simulink model "simulink5ms_plotAndGains"  (R2023a)
settings: Solver=ode3  StartTime=0.0  StopTime=1000  FixedStep=.001  RelTol=1e-3  EnableMultiTasking=on
undefined symbols (not defined in the file or in its folder): Serial_Port, Standard_Devices
libraries: sldrtlib x2
settings Model: SimulationMode=external  ExtModeTrigDuration=10000  Creator=d-block  LastModifiedBy=rout3
settings SolverCC: AlgebraicLoopSolver=TrustRegion
settings DataIOCC: LimitDataPoints=on  SaveFormat=Array  ReturnWorkspaceOutputs=off
settings OptimizationCC: LifeSpan=inf
settings DebuggingCC: UnconnectedInputMsg=warning  UnconnectedOutputMsg=warning  UnconnectedLineMsg=warning  SFUnexpectedBacktrackingDiag=warning  SFNoUnconditionalDefaultTransitionDiag=warning  ArithmeticOperatorsInVariantConditions=warning
settings HardwareCC: ProdBitPerLong=64  ProdHWDeviceType=Intel->x86-64 (Linux 64)  TargetBitPerLong=64  TargetBitPerPointer=64  TargetIntDivRoundTo=Zero  TargetEndianess=LittleEndian  TargetWordSize=64  TargetHWDeviceType=Intel->x86-64
settings ModelReferenceCC: EnableRefExpFcnMdlSchedulingChecks=on  PropagateSignalLabelsOutOfModel=off
settings SFSimCC: SimUseLocalCustomCode=off  CustomCodeUndefinedFunction=UseInterfaceOnly
settings RTWCC: Description=Simulink Desktop Real-Time  SystemTargetFile=sldrt.tlc  TemplateMakefile=sldrt.tmf  RTWUseLocalCustomCode=off  RTWCompilerOptimization=on  DLArmComputeVersion=19.05
settings CodeAppCC: MaxIdLength=95  StateflowObjectComments=on
settings SimulinkDesktopRealTimeCC: TargetLibSuffix=_sldrt.a  TargetPreCompLibLocation=C:\MATLABR2023a\toolbox\sldrt\lib\win64  TargetLangStandard=C89/C90 (ANSI)  SupportVariableSizeSignals=off
settings ConfigComp: CovMetricSettings=dw  CovSaveCumulativeToWorkspaceVar=on  CovSaveSingleToWorkspaceVar=on  CovExternalEMLEnable=off

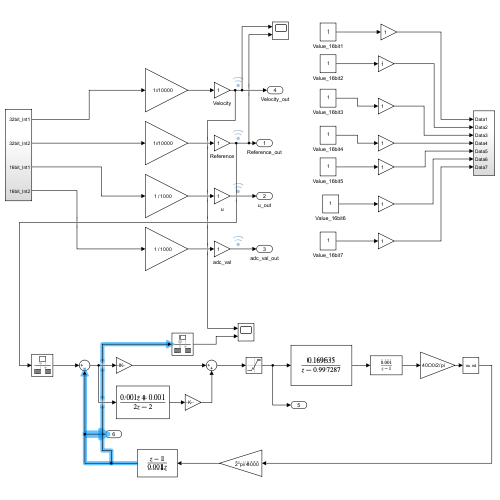
[thumbnail: Simulink's stored preview of the top-level diagram]
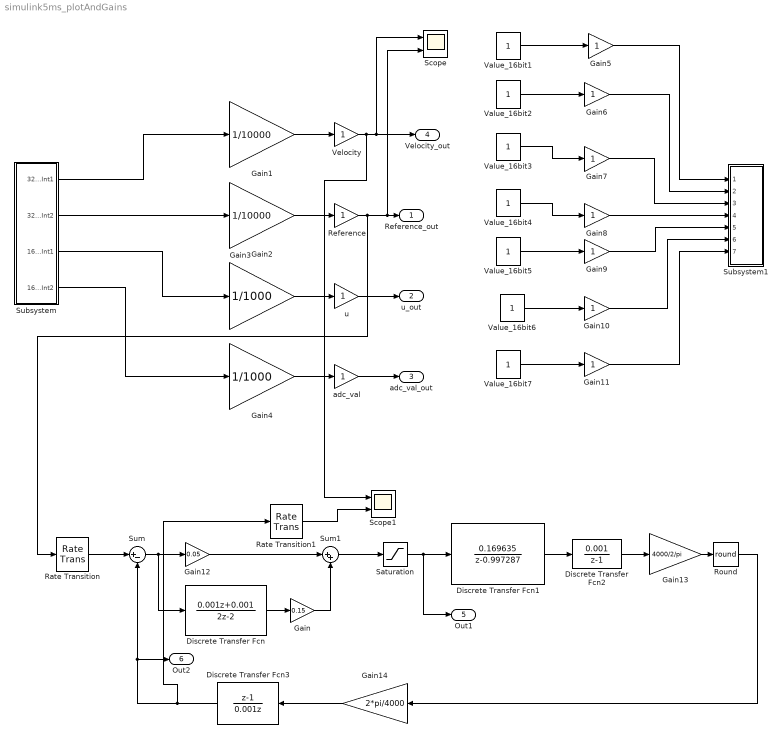
== system simulink5ms_plotAndGains ==
  Discrete Transfer Fcn : DiscreteTransferFcn  Numerator=[0.001 0.001]  Denominator=[2 -2]  SampleTime=0.001
  Discrete Transfer Fcn1 : DiscreteTransferFcn  Numerator=[0.169635]  Denominator=[1 -0.997287]  SampleTime=0.001
  Discrete Transfer Fcn2 : DiscreteTransferFcn  Numerator=[0.001]  Denominator=[1 -1]  SampleTime=0.001
  Discrete Transfer Fcn3 : DiscreteTransferFcn  Numerator=[1 -1]  Denominator=[0.001 0]  SampleTime=0.001
  Gain : Gain  Gain=0.15
  Gain1 : Gain  Gain=1/10000  OutDataTypeStr=double  SaturateOnIntegerOverflow=on  ParamDataTypeStr=Inherit: Same as input
  Gain{5..11} (7 alike) : Gain
  Gain12 : Gain  Gain=0.05
  Gain13 : Gain  Gain=4000/2/pi
  Gain14 : Gain  Gain=2*pi/4000
  Gain2 : Gain  Gain=1/10000  OutDataTypeStr=double  SaturateOnIntegerOverflow=on  ParamDataTypeStr=Inherit: Same as input
  Gain3 : Gain  Gain=1/1000  OutDataTypeStr=double  SaturateOnIntegerOverflow=on  ParamDataTypeStr=Inherit: Same as input
  Gain4 : Gain  Gain=1/1000  OutDataTypeStr=double  SaturateOnIntegerOverflow=on  ParamDataTypeStr=Inherit: Same as input
  Rate Transition : RateTransition  OutPortSampleTime=0.001
  Rate Transition1 : RateTransition  OutPortSampleTime=0.005
  Reference : Gain
  Round : Rounding  Operator=round
  Saturation : Saturate  UpperLimit=10  LowerLimit=-10
  Scope : Scope  NumInputPorts=2
  Scope1 : Scope  NumInputPorts=2
  Subsystem : Subsystem
  Subsystem1 : Subsystem
  Sum : Sum  Inputs=|+-
  Sum1 : Sum  Inputs=|++
  Value_16bit{1..4,6..7} (6 alike) : Constant
  "Value_16bit5 " : Constant
  Velocity : Gain
  adc_val : Gain
  u : Gain
  Reference_out : Outport
  u_out : Outport  Port=2
  adc_val_out : Outport  Port=3
  Velocity_out : Outport  Port=4
  Out1 : Outport  Port=5
  Out2 : Outport  Port=6
  wires:
  Gain2/1 -> Reference/1
  Value_16bit2/1 -> Gain6/1
  Value_16bit3/1 -> Gain7/1
  Value_16bit4/1 -> Gain8/1
  "Value_16bit5 "/1 -> Gain9/1
  Subsystem/3(16bit_Int1) -> Gain3/1
  Subsystem/4(16bit_Int2) -> Gain4/1
  Subsystem/2(32bit_Int2) -> Gain2/1
  Value_16bit1/1 -> Gain5/1
  Value_16bit6/1 -> Gain10/1
  Value_16bit7/1 -> Gain11/1
  Gain5/1 -> Subsystem1/1(Data1)
  Gain6/1 -> Subsystem1/2(Data2)
  Gain7/1 -> Subsystem1/3(Data3)
  Gain8/1 -> Subsystem1/4(Data4)
  Gain9/1 -> Subsystem1/5(Data5)
  Gain10/1 -> Subsystem1/6("Data6 ")
  Gain11/1 -> Subsystem1/7("Data7 ")
  Gain3/1 -> u/1
  Gain4/1 -> adc_val/1
  Reference/1 -> Rate Transition/1, Scope/2, Reference_out/1
  u/1 -> u_out/1
  adc_val/1 -> adc_val_out/1
  Velocity/1 -> Scope1/1, Scope/1, Velocity_out/1
  Gain1/1 -> Velocity/1
  Subsystem/1(32bit_Int1) -> Gain1/1
  Discrete Transfer Fcn3/1 -> Rate Transition1/1, Sum/2, Out2/1
  Round/1 -> Gain14/1
  Discrete Transfer Fcn1/1 -> Discrete Transfer Fcn2/1
  Gain12/1 -> Sum1/1
  Sum/1 -> Discrete Transfer Fcn/1, Gain12/1
  Gain13/1 -> Round/1
  Saturation/1 -> Out1/1, Discrete Transfer Fcn1/1
  Gain/1 -> Sum1/2
  Sum1/1 -> Saturation/1
  Discrete Transfer Fcn/1 -> Gain/1
  Gain14/1 -> Discrete Transfer Fcn3/1
  Discrete Transfer Fcn2/1 -> Gain13/1
  Rate Transition/1 -> Sum/1
  Rate Transition1/1 -> Scope1/2

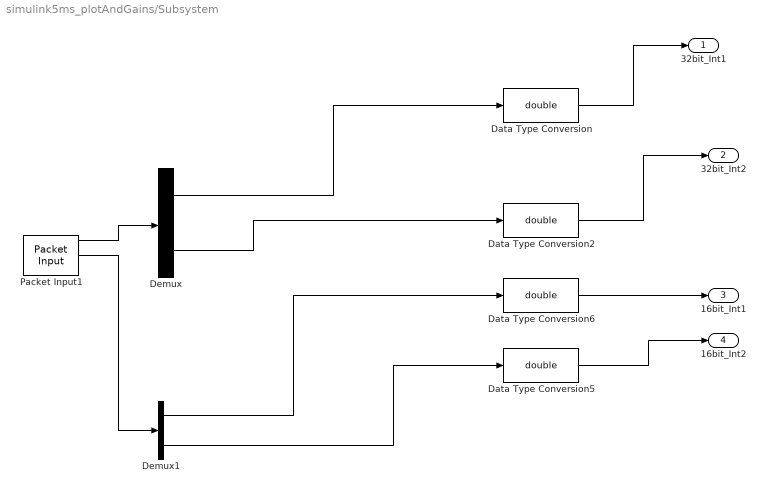
== system simulink5ms_plotAndGains/Subsystem ==
  Data Type Conversion{,2,5..6} (4 alike) : DataTypeConversion  OutDataTypeStr=double  SaturateOnIntegerOverflow=off  RndMeth=Floor
  Demux : Demux  Outputs=2
  Demux1 : Demux  Outputs=2
  Packet Input1 : sldrtlib/Packet Input  SampleTime=.005  MaxMissedTicks=50  ShowMissedTicks=on  YieldWhenWaiting=off  DrvName=Standard_Devices/Serial_Port  DrvAddress=1  DrvOptions=[115200 8 0 0 0 0 0 1]  PacketSize=12  DataTypes={'2*int32','2*int16'}  ShowReady=off  ShowError=off  PacketID=1  ByteOrder=1  ShowTimestamp=off
      settings: AttributesFormatString=Serial Port [1]
  32bit_Int1 : Outport  VectorParamsAs1DForOutWhenUnconnected=off
  32bit_Int2 : Outport  Port=2  VectorParamsAs1DForOutWhenUnconnected=off
  16bit_Int1 : Outport  Port=3  VectorParamsAs1DForOutWhenUnconnected=off
  16bit_Int2 : Outport  Port=4  VectorParamsAs1DForOutWhenUnconnected=off
  wires:
  Data Type Conversion/1 -> 32bit_Int1/1
  Data Type Conversion2/1 -> 32bit_Int2/1
  Data Type Conversion6/1 -> 16bit_Int1/1
  Data Type Conversion5/1 -> 16bit_Int2/1
  Demux1/2 -> Data Type Conversion5/1
  Demux1/1 -> Data Type Conversion6/1
  Packet Input1/1 -> Demux/1
  Packet Input1/2 -> Demux1/1
  Demux/1 -> Data Type Conversion/1
  Demux/2 -> Data Type Conversion2/1

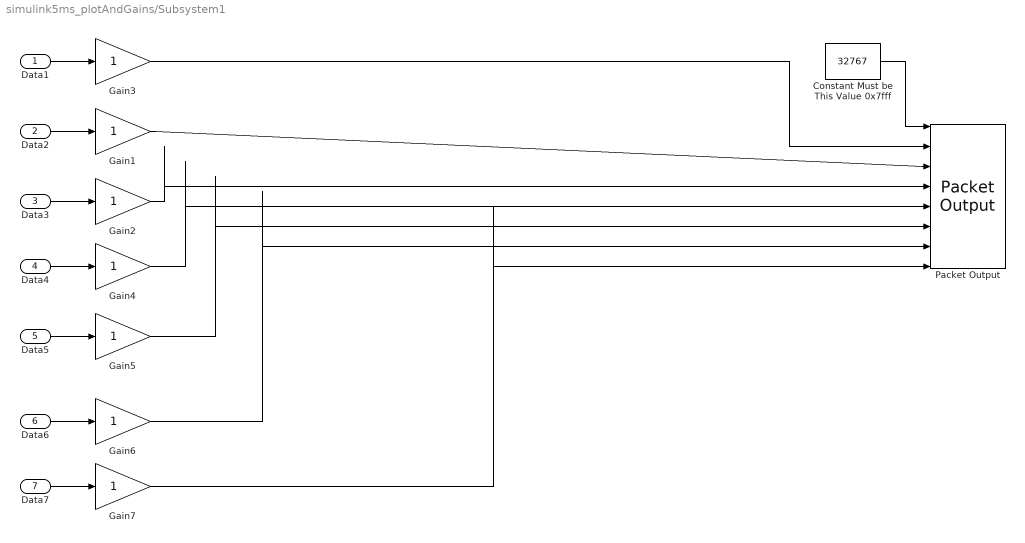
== system simulink5ms_plotAndGains/Subsystem1 ==
  Data1 : Inport
  Data2 : Inport  Port=2
  Data3 : Inport  Port=3
  Data4 : Inport  Port=4
  Data5 : Inport  Port=5
  "Data6 " : Inport  Port=6
  "Data7 " : Inport  Port=7
  Constant Must be This Value 0x7fff : Constant  Value=32767  OutDataTypeStr=int16
  Gain{1..7} (7 alike) : Gain  OutDataTypeStr=int16
  Packet Output : sldrtlib/Packet Output  SampleTime=.005  MaxMissedTicks=10  ShowMissedTicks=off  YieldWhenWaiting=off  DrvName=Standard_Devices/Serial_Port  DrvAddress=1  DrvOptions=[115200 8 0 0 0 0 0 1]  PacketSize=16  DataTypes={'int16','int16','int16','int16','int16','int16','int16','int16'}  ShowReady=off  ShowError=off  PacketID=1  ByteOrder=1  InitialValue=[]  FinalValue=[]
      settings: AttributesFormatString=Serial Port [1]
  wires:
  Data1/1 -> Gain3/1
  Data2/1 -> Gain1/1
  Data3/1 -> Gain2/1
  Data5/1 -> Gain5/1
  Gain3/1 -> Packet Output/2
  Data4/1 -> Gain4/1
  "Data6 "/1 -> Gain6/1
  "Data7 "/1 -> Gain7/1
  Constant Must be This Value 0x7fff/1 -> Packet Output/1
  Gain1/1 -> Packet Output/3
  Gain2/1 -> Packet Output/4
  Gain4/1 -> Packet Output/5
  Gain5/1 -> Packet Output/6
  Gain6/1 -> Packet Output/7
  Gain7/1 -> Packet Output/8
